simulink library "mpc555tpu"  (Simulink 6.0)
settings: Solver=ode45  SolverMode=SingleTasking  StartTime=0.0  StopTime=10.0  RelTol=1e-3
libraries: driver_interface_library x9, simulink x4
settings Model: Creator=The MathWorks Inc.  LastModifiedBy=batserve  ExtModeAutoUpdateStatusClock=off
settings OptimizationCC: BooleanDataType=off
settings DebuggingCC: CheckExecutionContextPreStartOutputMsg=on  CheckExecutionContextRuntimeOutputMsg=on  SolverPrmCheckMsg=none
settings HardwareCC: TargetUnknown=on

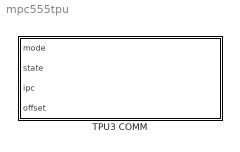
== system mpc555tpu ==
  TPU3 COMM : Subsystem  PropExecContextAcrossSSBoundary=on  mask(COMM (TPU3) Sensorles Mode){module=A, master_channel=0, master_channel_priority=Low, parameter_type=Channel and Parameter Index, counter_channel=0, counter_parameter=0, counter_parameter_name=brad, state_matrix={ 33 '100' 33 '010' 33 '001'  }, update_period=1}
      mask prompts: module "TPU module:"; master_channel "TPU master channel number:"; master_channel_priority "Master channel priority:"; parameter_type "Specify Counter Location By:"; counter_channel "Counter  Channel:"; counter_parameter "Counter  Channel Parameter (16bit ):"; counter_parameter_name "Counter  Alias:"; state_matrix "State Matrix:"; update_period "Update Period:"
      mask help:
      | Multiphase Motor Commutation TPU Function
      |
      | Input Ports
      | ---------------
      | mode:
      | 	0 	-	startup
      | 	1	-	run free
      |
      | state:
      | 	If mode is 'startup' then force the state to one of the states in the state
      | 	matrix. Index is 1 based.
      |
      | ipc:
      | 	Initial Position Counter. This value should be latched by the
      | 	NITC (TPU3) function. Used to synchronize the position
      | 	counter with the COMM. When the mode is transitioned from
      | 	startup to run this value is assumed to be in the middle of the
      | 	current state.
      |
      | offset:
      | 	During run time the CPU can increase offset to increase
      | 	torque. During the run mode it is advisable to set the
      | 	offset to be about 1.5 * the state length.
      mask init:
      | % check the alias parameter is not empty
      | if parameter_type == 2
      | 	counter_parameter_name = strtrim(counter_parameter_name);
      | 	if isempty(counter_parameter_name)
      | 		error(sprintf('\n"Counter Parameter Name" parameter cannot be empty'));
      | 	end
      | end
      | 
      | % Make master_channel 0 based
      | master_channel = master_channel - 1;
      | 
      | % Calculate the number of states
      | slen = length(state_matrix);
      | if rem(slen,2) ~= 0
      | 	error('The state matrix is badly formatted');
      | end
      | num_states = slen / 2;
      | 
      | % Validate the state matrix
      | num_pins = -1;
      | for i = 1:num_states
      | 	state_length = state_matrix{2*i-1};
      | 	state_pattern = state_matrix{2*i};
      | 	if ~regexp(state_pattern, '^(1|0)*$');
      | 		error('The state matrix is badly formatted');
      | 	end
      | 	if num_pins < 0
      | 		num_pins = length(state_pattern);
      | 	else
      | 		if num_pins ~= length(state_pattern);
      | 			error('The state matrix is badly formatted');
      | 		end
      | 	end
      | end
      mask StyleString: popup(A|B),popup(0|1|2|3|4|5|6|7|8|9|10|11|12|13|14|15),popup(Low|Medium|High),popup(Channel and Parameter Index|Parameter Alias),popup(0|1|2|3|4|5|6|7|8|9|10|12|13|14|15),popup(0|1|2|3|4|5|6|7|8|9|10|11|12|13|14|15),edit,edit,edit
      mask CallbackString:
      | |||switch get_param(gcb,'parameter_type')
      | 	case 'Channel and Parameter Index'
      | 		simUtil_maskParam('hide',gcb,'counter_parameter_name');
      | 		simUtil_maskParam('show',gcb,'counter_channel');
      | 		simUtil_maskParam('show',gcb,'counter_parameter');
      | 	case 'Parameter Alias'
      | 		simUtil_maskParam('show',gcb,'counter_parameter_name');
      | 		simUtil_maskParam('hide',gcb,'counter_channel');
      | 		simUtil_maskParam('hide',gcb,'counter_parameter');
      | 	otherwise
      | 		error(get_param(gcb,'parameter_type'));
      | end
      | ||||% State matrix example
      | % { 33 '100' 33 '010' 33 '001' }|
      mask Display: disp('COMM\n(TPU3)');

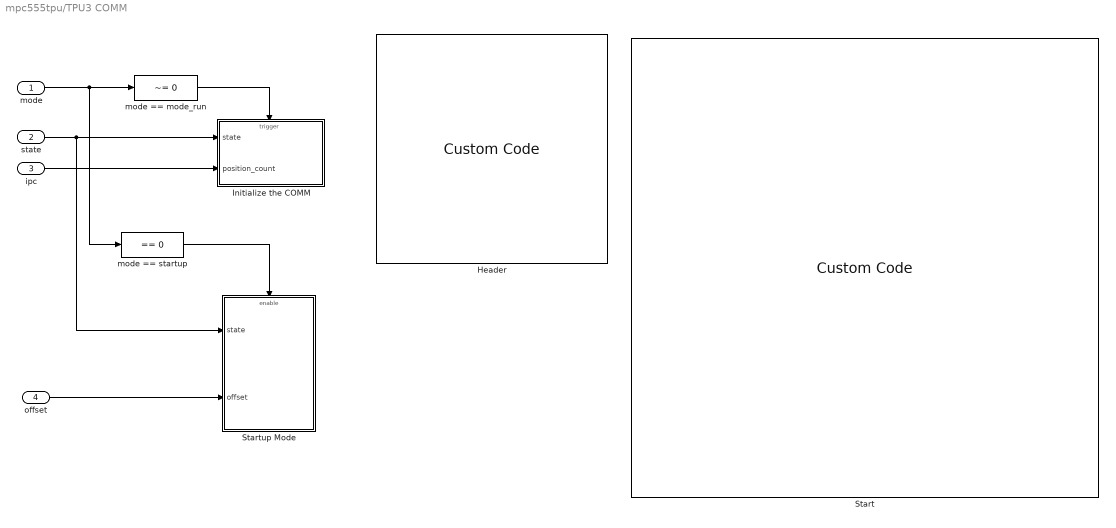
== system mpc555tpu/TPU3 COMM ==
  mode : Inport  Port=1  LatchInput=off
  state : Inport  Port=2  LatchInput=off
  ipc : Inport  Port=3  LatchInput=off
  offset : Inport  Port=4  LatchInput=off
  Header : driver_interface_library/Custom Code
  Initialize the COMM : Subsystem  PropExecContextAcrossSSBoundary=on
  Start : driver_interface_library/Custom Code
  Startup Mode : Subsystem  TreatAsAtomicUnit=on  PropExecContextAcrossSSBoundary=on
  mode == mode_run : simulink/Math Operations/Logic Operations/Compare To Constant  relop=~=  const=0  LogicOutDataTypeMode=uint8
  mode == startup : simulink/Math Operations/Logic Operations/Compare To Constant  relop===  const=0  LogicOutDataTypeMode=uint8
  wires:
  state/1 -> Initialize the COMM/1(state), Startup Mode/1(state)
  ipc/1 -> Initialize the COMM/2(position_count)
  mode/1 -> mode == mode_run/1, mode == startup/1
  mode == mode_run/1 -> Initialize the COMM/Trigger
  mode == startup/1 -> Startup Mode/Enable
  offset/1 -> Startup Mode/2(offset)

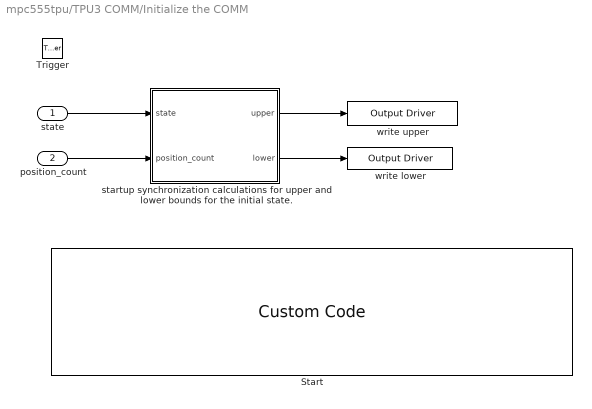
== system mpc555tpu/TPU3 COMM/Initialize the COMM ==
  state : Inport  Port=1  LatchInput=off
  position_count : Inport  Port=2  LatchInput=off
  Trigger : TriggerPort  ZeroCross=off
  Start : driver_interface_library/Custom Code
  startup synchronization calculations for upper and lower bounds for the initial state. : Subsystem  PropExecContextAcrossSSBoundary=on
  write lower : driver_interface_library/Output Driver  operation_type=LHS Assignment  input_is_contiguous=off  t=-1  expr=sprintf('TPU_%s.PARM.R[%d][5]', module, master_channel)  port_width=1  pOpt=[]
  write upper : driver_interface_library/Output Driver  operation_type=LHS Assignment  input_is_contiguous=off  t=-1  expr=sprintf('TPU_%s.PARM.R[%d][4]', module, master_channel)  port_width=1  pOpt=[]
  wires:
  startup synchronization calculations for upper and lower bounds for the initial state./1(upper) -> write upper/1
  startup synchronization calculations for upper and lower bounds for the initial state./2(lower) -> write lower/1
  state/1 -> startup synchronization calculations for upper and lower bounds for the initial state./1(state)
  position_count/1 -> startup synchronization calculations for upper and lower bounds for the initial state./2(position_count)

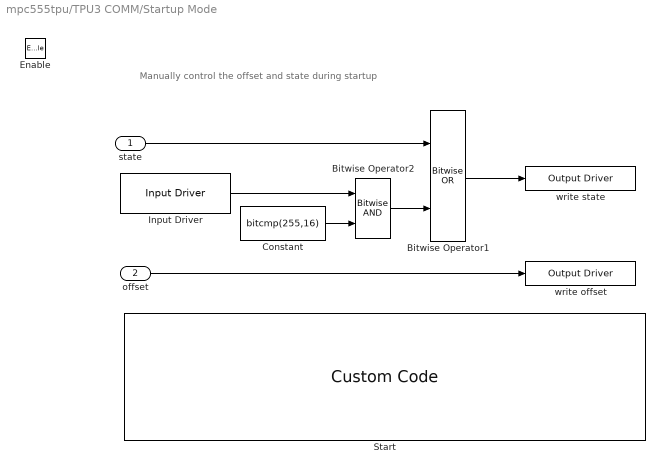
== system mpc555tpu/TPU3 COMM/Startup Mode ==
  note: Manually control the offset and state during startup
  state : Inport  Port=1  DataType=uint16  LatchInput=off
  offset : Inport  Port=2  DataType=uint16  LatchInput=off
  Enable : EnablePort
  Bitwise Operator1 : simulink/Bit Operations/Bitwise Operator  logicop=OR  UseBitMask=off  NumInputPorts=2  BitMask=bin2dec('11011001')  BitMaskRealWorld=Stored Integer
  Bitwise Operator2 : simulink/Bit Operations/Bitwise Operator  logicop=AND  UseBitMask=off  NumInputPorts=2  BitMask=bin2dec('11011001')  BitMaskRealWorld=Stored Integer
  Constant : Constant  Value=bitcmp(255,16)  OutDataTypeMode=uint16
  Input Driver : driver_interface_library/Input Driver  t=-1  expr=sprintf('TPU_%s.PARM.R[%d][1]', module, master_channel)  portWidth=1  pOpt=[]  expression_type=Expression
  Start : driver_interface_library/Custom Code
  write offset : driver_interface_library/Output Driver  operation_type=LHS Assignment  input_is_contiguous=off  t=-1  expr=sprintf('TPU_%s.PARM.R[%d][2]', module, master_channel)  port_width=1  pOpt=[]
  write state : driver_interface_library/Output Driver  operation_type=LHS Assignment  input_is_contiguous=off  t=-1  expr=sprintf('TPU_%s.PARM.R[%d][1]', module, master_channel)  port_width=1  pOpt=[]
  wires:
  Input Driver/1 -> Bitwise Operator2/1
  Constant/1 -> Bitwise Operator2/2
  Bitwise Operator2/1 -> Bitwise Operator1/2
  state/1 -> Bitwise Operator1/1
  Bitwise Operator1/1 -> write state/1
  offset/1 -> write offset/1

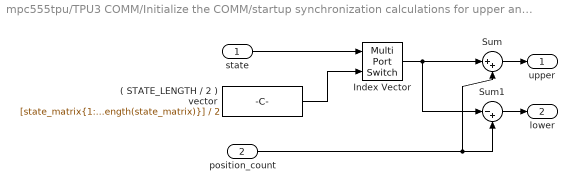
== system mpc555tpu/TPU3 COMM/Initialize the COMM/startup synchronization calculations for upper and lower bounds for the initial state. ==
  state : Inport  Port=1  LatchInput=off
  position_count : Inport  Port=2  LatchInput=off
  ( STATE_LENGTH / 2 ) vector : Constant  Value=[state_matrix{1:2:length(state_matrix)}] / 2
  Index Vector : MultiPortSwitch  Inputs=1
  Sum : Sum  Inputs=|++  SaturateOnIntegerOverflow=on
  Sum1 : Sum  Inputs=|-+  SaturateOnIntegerOverflow=on
  upper : Outport
  lower : Outport  Port=2
  wires:
  Index Vector/1 -> Sum/1, Sum1/1
  position_count/1 -> Sum/2, Sum1/2
  ( STATE_LENGTH / 2 ) vector/1 -> Index Vector/2
  state/1 -> Index Vector/1
  Sum/1 -> upper/1
  Sum1/1 -> lower/1
